simulink model "rlwatertank"  (R2022b)
settings: Solver=FixedStepAuto  StartTime=0.0  StopTime=200.0  FixedStep=0.01  RelTol=1e-3  EnableMultiTasking=on
undefined symbols (not defined in the file): DiscIntNeverNeededParam
settings Model: DataDictionary=BusSystem.sldd  Creator=The MathWorks, Inc.  LastModifiedBy=Robert
settings SolverCC: AlgebraicLoopSolver=TrustRegion
settings DataIOCC: LimitDataPoints=on  SaveOutput=off  ReturnWorkspaceOutputs=off  SignalLoggingName=logsOut
settings OptimizationCC: ExpressionDepthLimit=2147483647  InitFltsAndDblsToZero=on  LifeSpan=inf
settings DebuggingCC: SaveWithParameterizedLinksMsg=none  UnderspecifiedInitializationDetection=Classic  MergeDetectMultiDrivingBlocksExec=none  SignalResolutionControl=TryResolveAllWithWarning  MultiTaskDSMMsg=warning  FcnCallInpInsideContextMsg=warning  UnconnectedInputMsg=warning  UnconnectedOutputMsg=warning  UnconnectedLineMsg=warning  AllowSymbolicDim=off  StateNameClashWarn=warning  SFUnexpectedBacktrackingDiag=warning  SFNoUnconditionalDefaultTransitionDiag=warning  SFExecutionAtInitializationDiag=none  SFMachineParentedDataDiag=warning  ArithmeticOperatorsInVariantConditions=warning
settings HardwareCC: ProdBitPerPointer=32  ProdBitPerSizeT=32  ProdBitPerPtrDiffT=32  ProdLargestAtomicFloat=None  ProdIntDivRoundTo=Undefined  ProdEndianess=Unspecified  ProdWordSize=32  ProdHWDeviceType=Specified
settings ModelReferenceCC: EnableRefExpFcnMdlSchedulingChecks=on  PropagateSignalLabelsOutOfModel=off
settings SFSimCC: SimUseLocalCustomCode=off  CustomCodeUndefinedFunction=UseInterfaceOnly
settings RTWCC: RTWUseLocalCustomCode=off  DLArmComputeVersion=19.05
settings CodeAppCC: StateflowObjectComments=on
settings GRTTargetCC: TargetFcnLib=ansi_tfl_tmw.mat  TargetLangStandard=C89/C90 (ANSI)  CombineOutputUpdateFcns=off  GRTInterface=on
settings ConfigComp: CovMetricSettings=dw  CovSaveCumulativeToWorkspaceVar=on  CovSaveSingleToWorkspaceVar=on  CovExternalEMLEnable=off

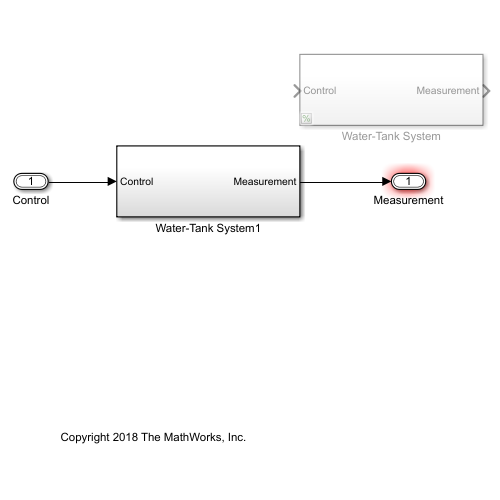
[thumbnail: Simulink's stored preview of the top-level diagram]
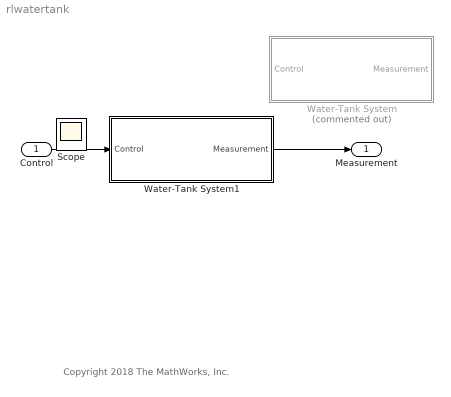
== system rlwatertank ==
  note: Copyright 2018 The MathWorks, Inc.
  Control : Inport  OutDataTypeStr=Bus: Control
  Water-Tank System : Subsystem  Commented=on
  Water-Tank System1 : Subsystem
  Measurement : Outport  OutDataTypeStr=Bus: slBus3
  Scope : Scope
  wires:
  Control/1 -> Water-Tank System1/1(Control)
  Water-Tank System1/1(Measurement) -> Measurement/1

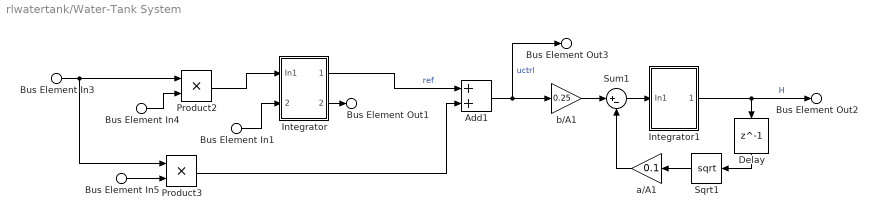
== system rlwatertank/Water-Tank System ==
  Bus Element In3 : Inport  PortName=Control  Element=Error
  Bus Element In4 : Inport  PortName=Control  Element=KI
  Bus Element In5 : Inport  PortName=Control  Element=KP
  Bus Element In1 : Inport  PortName=Control  Element=Iprev
  Add1 : Sum
  Delay : Delay  DelayLength=1
  Integrator : Subsystem
  Integrator1 : Subsystem
  Product2 : Product
  Product3 : Product
  Sqrt1 : Sqrt  OutputSignalType=real
  Sum1 : Sum  Inputs=|+-  SaturateOnIntegerOverflow=on
  a/A1 : Gain  Gain=0.1  SaturateOnIntegerOverflow=on  OutDataTypeStr=Inherit: Same as input  ParamDataTypeStr=Inherit: Same as input
  b/A1 : Gain  Gain=0.25  SaturateOnIntegerOverflow=on  OutDataTypeStr=Inherit: Same as input  ParamDataTypeStr=Inherit: Same as input
  Bus Element Out2 : Outport  PortName=Measurement  Element=Height
  Bus Element Out3 : Outport  PortName=Measurement  Element=uctrl
  Bus Element Out1 : Outport  PortName=Measurement  Element=Inext
  wires:
  Integrator/1(Out1) -> Add1/1  "ref"
  Add1/1 -> Bus Element Out3/1, b/A1/1  "uctrl"
  Integrator1/1(Out1) -> Bus Element Out2/1, Delay/1  "H"
  a/A1/1 -> Sum1/2
  Bus Element In3/1 -> Product3/1, Product2/1
  Product3/1 -> Add1/2
  Sqrt1/1 -> a/A1/1
  b/A1/1 -> Sum1/1
  Bus Element In4/1 -> Product2/2
  Sum1/1 -> Integrator1/1(In1)
  Product2/1 -> Integrator/1(In1)
  Bus Element In5/1 -> Product3/2
  Delay/1 -> Sqrt1/1
  Bus Element In1/1 -> Integrator/2(Iprev)
  Integrator/2(Inext) -> Bus Element Out1/1

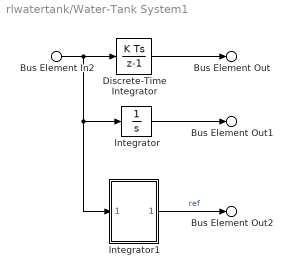
== system rlwatertank/Water-Tank System1 ==
  Bus Element In2 : Inport  PortName=Control  Element=Input
  Discrete-Time Integrator : DiscreteIntegrator  SampleTime=-1  ICPrevOutput=DiscIntNeverNeededParam  ICPrevScaledInput=DiscIntNeverNeededParam
  Integrator : Integrator
  Integrator1 : Subsystem
  Bus Element Out : Outport  PortName=Measurement  Element=Discrete
  Bus Element Out1 : Outport  PortName=Measurement  Element=Cont
  Bus Element Out2 : Outport  PortName=Measurement  Element=Own
  wires:
  Bus Element In2/1 -> Integrator1/1(Control), Integrator/1, Discrete-Time Integrator/1
  Discrete-Time Integrator/1 -> Bus Element Out/1
  Integrator/1 -> Bus Element Out1/1
  Integrator1/1(Measurement) -> Bus Element Out2/1  "ref"

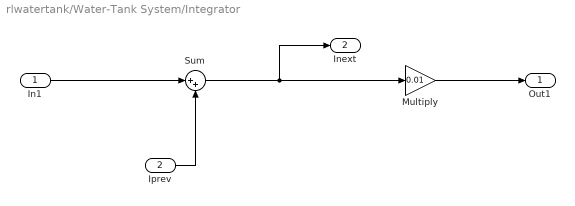
== system rlwatertank/Water-Tank System/Integrator ==
  In1 : Inport
  Iprev : Inport  Port=2
  Multiply : Gain  Gain=0.01
  Sum : Sum  Inputs=|++
  Out1 : Outport
  Inext : Outport  Port=2
  wires:
  In1/1 -> Sum/1
  Multiply/1 -> Out1/1
  Sum/1 -> Inext/1, Multiply/1
  Iprev/1 -> Sum/2

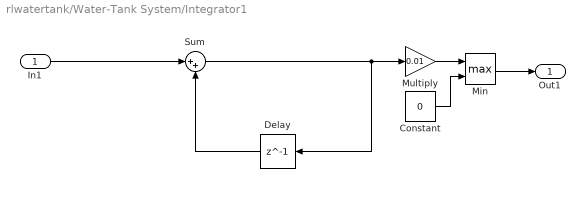
== system rlwatertank/Water-Tank System/Integrator1 ==
  In1 : Inport
  Constant : Constant  Value=0
  Delay : Delay  DelayLength=1
  Min : MinMax  Function=max  Inputs=2
  Multiply : Gain  Gain=0.01
  Sum : Sum  Inputs=|++
  Out1 : Outport
  wires:
  Delay/1 -> Sum/2
  Sum/1 -> Multiply/1, Delay/1
  Multiply/1 -> Min/1
  Min/1 -> Out1/1
  Constant/1 -> Min/2
  In1/1 -> Sum/1

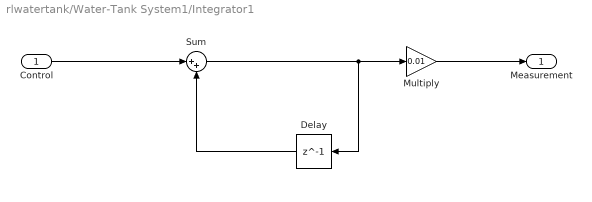
== system rlwatertank/Water-Tank System1/Integrator1 ==
  Control : Inport
  Delay : Delay  DelayLength=1
  Multiply : Gain  Gain=0.01
  Sum : Sum  Inputs=|++
  Measurement : Outport
  wires:
  Control/1 -> Sum/1
  Delay/1 -> Sum/2
  Sum/1 -> Delay/1, Multiply/1
  Multiply/1 -> Measurement/1
